simulink model "subsystem"  (R2022a)
settings: Solver=VariableStepAuto  StartTime=0.0  StopTime=10.0  RelTol=1e-3
settings Model: Creator=Jagadeesh  LastModifiedBy=Jagadeesh

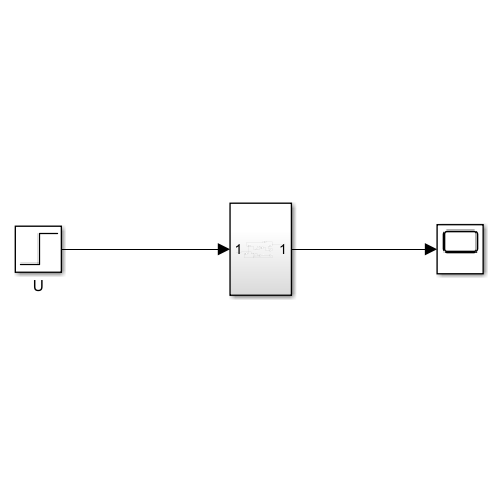
[thumbnail: Simulink's stored preview of the top-level diagram]
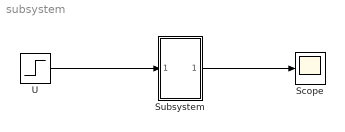
== system subsystem ==
  Scope : Scope
  Subsystem : Subsystem
  U : Step  SampleTime=0
  wires:
  U/1 -> Subsystem/1(In1)
  Subsystem/1(Out1) -> Scope/1

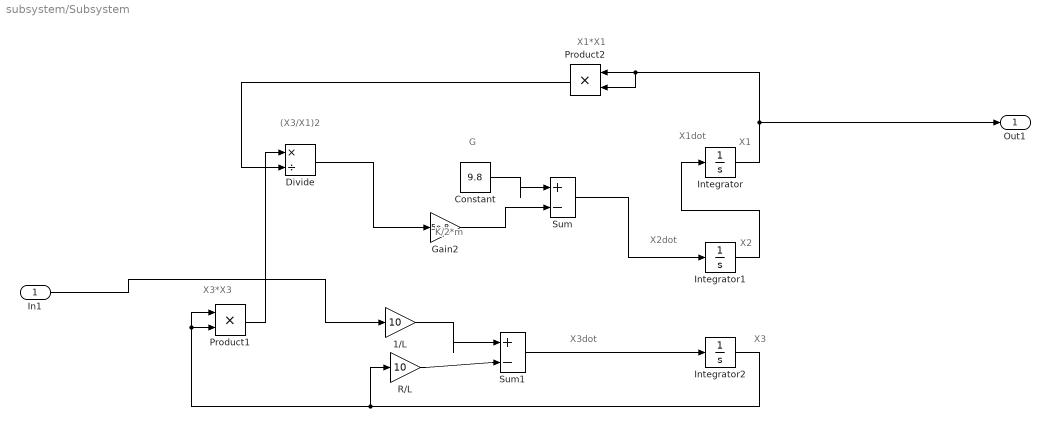
== system subsystem/Subsystem ==
  note: K/2*m
  note: G
  note: X3*X3
  note: (X3/X1)2
  note: X1*X1
  note: X1
  note: X1dot
  note: X2
  note: X2dot
  note: X3
  note: X3dot
  In1 : Inport
  1/L : Gain  Gain=10
  Constant : Constant  Value=9.8
  Divide : Product  Inputs=*/
  Gain2 : Gain  Gain=5e-8
  Integrator : Integrator
  Integrator1 : Integrator
  Integrator2 : Integrator
  Product1 : Product
  Product2 : Product
  R/L : Gain  Gain=10
  Sum : Sum  Inputs=|+-
  Sum1 : Sum  Inputs=|+-
  Out1 : Outport
  wires:
  1/L/1 -> Sum1/1
  Integrator2/1 -> Product1/2, Product1/1, R/L/1
  Constant/1 -> Sum/1
  Integrator1/1 -> Integrator/1
  Product1/1 -> Divide/1
  Gain2/1 -> Sum/2
  R/L/1 -> Sum1/2
  Integrator/1 -> Out1/1, Product2/2, Product2/1
  Sum1/1 -> Integrator2/1
  Product2/1 -> Divide/2
  Divide/1 -> Gain2/1
  Sum/1 -> Integrator1/1
  In1/1 -> 1/L/1
